simulink subsystem "Real_Derivative"  (R2022b)
settings: Solver=VariableStepAuto  StartTime=0.0  StopTime=10.0  RelTol=1e-3
libraries: simulink x1
settings Model: Creator=gotta  LastModifiedBy=gotta

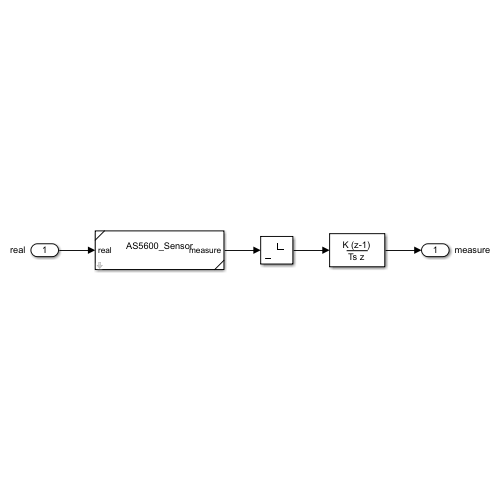
[thumbnail: Simulink's stored preview of the top-level diagram]
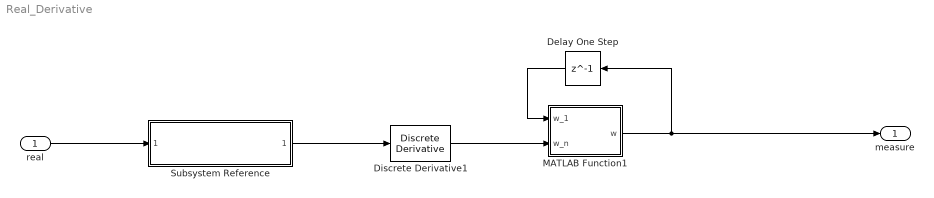
== system Real_Derivative ==
  real : Inport
  Delay One Step : Delay  DelayLength=1
  Discrete Derivative1 : simulink/Discrete/Discrete Derivative  gainval=1.0  ICPrevScaledInput=0.0  OutMin=[]  OutMax=[]  OutDataType=fixdt(1, 16)  OutScaling=2^-10  DoSatur=off
  MATLAB Function1 : MATLAB Function  TreatAsAtomicUnit=on
  Subsystem Reference : Subsystem  ReferencedSubsystem=AS5600_Sensor  sensor_model=AS5600  wrapping=off  offset=0
  measure : Outport
  wires:
  Delay One Step/1 -> MATLAB Function1/1(w_1)
  real/1 -> Subsystem Reference/1
  MATLAB Function1/1(w) -> Delay One Step/1, measure/1
  Discrete Derivative1/1 -> MATLAB Function1/2(w_n)
  Subsystem Reference/1 -> Discrete Derivative1/1

== matlab function Real_Derivative/MATLAB Function1 ==
  data: w_1 input; w output; w_n input
function w = fcn(w_1, w_n)

if abs(w_n-w_1) > 100
    w = w_1;
else
    w = w_n;
end
